simulink model "chap1_1"  (R2023b)
settings: Solver=ode45  StartTime=0.0  StopTime=10.0  RelTol=1e-3
settings Model: Creator=CorgiQvm  LastModifiedBy=CorgiQvm

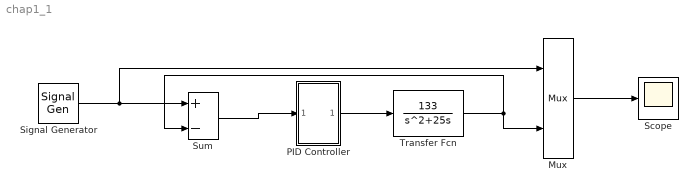
== system chap1_1 ==
  Mux : Mux  Inputs=2
  PID Controller : Subsystem  mask{P=60, I=1, D=3}
      mask prompts: P "Proportional"; I "Integral"; D "Derivative"
      mask DialogControl ParameterGroupVar Prompt: 参数
      mask Display: disp('PID');
  Scope : Scope
  Signal Generator : SignalGenerator  Frequency=0.2
  Sum : Sum  Inputs=+-  InputSameDT=on  SaturateOnIntegerOverflow=on  OutDataTypeStr=Inherit: Same as first input
  Transfer Fcn : TransferFcn  Numerator=[133]  Denominator=[1 25 0]
  wires:
  Signal Generator/1 -> Mux/1, Sum/1
  Sum/1 -> PID Controller/1(In1)
  PID Controller/1(Out1) -> Transfer Fcn/1
  Transfer Fcn/1 -> Mux/2, Sum/2
  Mux/1 -> Scope/1

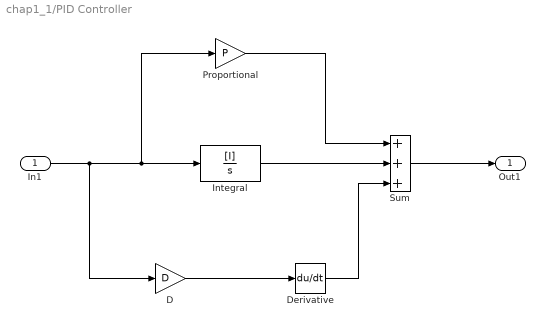
== system chap1_1/PID Controller ==
  In1 : Inport
  D : Gain  Gain=D  SaturateOnIntegerOverflow=on  OutDataTypeStr=Inherit: Same as input  ParamDataTypeStr=Inherit: Same as input
  Derivative : Derivative
  Integral : TransferFcn  Numerator=[I]  Denominator=[1 0]
  Proportional : Gain  Gain=P  SaturateOnIntegerOverflow=on  OutDataTypeStr=Inherit: Same as input  ParamDataTypeStr=Inherit: Same as input
  Sum : Sum  Inputs=+++  InputSameDT=on  SaturateOnIntegerOverflow=on  OutDataTypeStr=Inherit: Same as first input
  Out1 : Outport
  wires:
  D/1 -> Derivative/1
  Integral/1 -> Sum/2
  Proportional/1 -> Sum/1
  In1/1 -> D/1, Proportional/1, Integral/1
  Sum/1 -> Out1/1
  Derivative/1 -> Sum/3
